simulink model "Vehicle_definitivo_validazione_2"  (R2025b)
settings: Solver=ode4  StartTime=0.0  StopTime=30  FixedStep=0.001  RelTol=1e-3
undefined symbols (not defined in the file): car, new_lotus_bump, new_lotus_roll, new_lotus_steer, posRef, rad, s, Tau_1, Tau_2, Tau_3, Tau_4, yawRef
libraries: aerolibconvert2 x28, simulink_extras x16, simulink x12, slpidlib x2, mpclib x1
(part 13 of 13)

== matlab function Vehicle_definitivo_validazione_2/Senza relaxation/Vehicle/Powertrain/Electric Motor/MATLAB Function ==
  data: T_FR input; T_FL input; w_FR input; w_FL input; SoC input; SoC_dot output
function SoC_dot  = fcn_Battery(T_FR, T_FL, w_FR, w_FL, SoC)
    
    % --- 1. PARAMETRI BATTERIA E POWERTRAIN ---
    C_Ah = 50; % Capacità totale del pacco batteria in Ah (es. accumulatore FS)
    n_cells_series = 100; % Numero di celle collegate in serie
    eta_em = 0.95; % Efficienza combinata Motore + Inverter
    P_aux = 500;   % [Watt] Potenza costantemente assorbita dai servizi (pompe, LV, ECU)
    
    % --- 2. CURVE CARATTERISTICHE (Dipendenti dal SoC) ---
    % Approssimazione lineare per cella Li-ion: da 3.0V (scarica) a 4.2V (carica)
    OCV_cell = 3.0 + (1.2 * SoC); 
    Rin_cell = 0.005; % Resistenza interna della singola cella [Ohm]
    
    V_oc = OCV_cell * n_cells_series; % Tensione a vuoto dell'intero pacco
    R_in = Rin_cell * n_cells_series; % Resistenza interna totale
    
    % --- 3. POTENZA ELETTRICA MOTORE 1 ---
    P_mech1 = T_FR * w_FR;
    if P_mech1 >= 0
        P_elec1 = P_mech1 / eta_em; % Trazione: assorbe più di quanto eroga
    else
        P_elec1 = P_mech1 * eta_em; % Rigenerazione: immette meno di quanto frena
    end
    
    % --- 4. POTENZA ELETTRICA MOTORE 2 ---
    P_mech2 = T_FL * w_FL;
    if P_mech2 >= 0
        P_elec2 = P_mech2 / eta_em; % Trazione
    else
        P_elec2 = P_mech2 * eta_em; % Rigenerazione
    end
    
    % --- 5. CARICO ELETTRICO TOTALE SULLA BATTERIA ---
    % La batteria vede la somma algebrica dei due inverter più i servizi
    P_tot_elec = P_elec1 + P_elec2 + P_aux;
    
    % --- 6. CALCOLO CORRENTE E TENSIONE (CIRCUITO EQUIVALENTE) ---
    % Risoluzione dell'equazione di 2° grado: Rin * I^2 - Voc * I + P_tot = 0
    discriminante = V_oc^2 - 4 * R_in * P_tot_elec;
    
    if discriminante < 0
        % Protezione numerica: la richiesta di potenza supera il limite fisico
        % della batteria (il voltage sag la manderebbe a zero). 
        % Eroga la corrente massima teorica (Cortocircuito).
        I_batt = V_oc / (2 * R_in); 
    else
        % Soluzione standard per la corrente prelevata (o immessa se P_tot < 0)
        I_batt = (V_oc - sqrt(discriminante)) / (2 * R_in);
    end
    
    % Voltaggio reale ai morsetti (al netto del Voltage Sag)
    V_batt = V_oc - R_in * I_batt;
    
    % Potenza dissipata per effetto Joule (utile per dimensionare il raffreddamento)
    P_dissipata = R_in * (I_batt^2);
    
    % --- 7. DERIVATA DELLO STATE OF CHARGE (Coulomb Counting) ---
    % SoC_dot [1/s]. I_batt è in Ampere (C/s), la capacità si porta in Coulomb (*3600)
    SoC_dot = -I_batt / (C_Ah * 3600);
    
end

== matlab function Vehicle_definitivo_validazione_2/Torque Vectoring/Vehicle/Solver/MATLAB Function ==
  data: Fx input; Fy input; toe input; u_dot output size=1; v_dot output size=1; drag input; car input; u input; v input; r input; yaw_rate_dot output size=1; ax output size=1; ay output size=1
function [u_dot, v_dot, yaw_rate_dot, ax, ay]   = fcn_Solver(Fx, Fy, toe, drag, car, u, v, r)

% --- Accelerazione Longitudinale (asse X veicolo) ---
u_dot = ( Fx(1)*cos(toe(1)) - Fy(1)*sin(toe(1)) + ...
          Fx(2)*cos(toe(2)) - Fy(2)*sin(toe(2)) + ...
          Fx(3)*cos(toe(3)) - Fy(3)*sin(toe(3)) + ...
          Fx(4)*cos(toe(4)) - Fy(4)*sin(toe(4)) - drag ) / car.m + v * r;

% --- Accelerazione Laterale (asse Y veicolo) ---
v_dot = ( Fx(1)*sin(toe(1)) + Fy(1)*cos(toe(1)) + ...
          Fx(2)*sin(toe(2)) + Fy(2)*cos(toe(2)) + ...
          Fx(3)*sin(toe(3)) + Fy(3)*cos(toe(3)) + ...
          Fx(4)*sin(toe(4)) + Fy(4)*cos(toe(4)) ) / car.m - u * r;

% --- Derivata del Rateo di Imbardata (attorno asse Z) ---
yaw_rate_dot = 1 / car.Izz * ( ...
    ... % Momento dalle forze laterali all'asse anteriore (+lf)
    (Fx(1)*sin(toe(1)) + Fy(1)*cos(toe(1)) + Fx(2)*sin(toe(2)) + Fy(2)*cos(toe(2))) * car.lf ...
    ... % Momento dalle forze laterali all'asse posteriore (-lr)
  - (Fx(3)*sin(toe(3)) + Fy(3)*cos(toe(3)) + Fx(4)*sin(toe(4)) + Fy(4)*cos(toe(4))) * car.lr ...
   ... % Momento dalla carreggiata anteriore (spinta asimmetrica dx/sx)
  - (Fx(2)*cos(toe(2)) - Fy(2)*sin(toe(2)) - Fx(1)*cos(toe(1)) + Fy(1)*sin(toe(1))) * car.tf / 2 ...
    ... % Momento dalla carreggiata posteriore (spinta asimmetrica dx/sx)
  - (Fx(4)*cos(toe(4)) - Fy(4)*sin(toe(4)) - Fx(3)*cos(toe(3)) + Fy(3)*sin(toe(3))) * car.tr / 2 );

% --- Accelerazioni nel sistema di riferimento ---
ax = u_dot - v * r;
ay = v_dot + u * r;

== matlab function Vehicle_definitivo_validazione_2/Torque Vectoring/Vehicle/Tyres/MATLAB Function ==
  data: Fx input; omega_dot output; Fz input; T_motor input; J input; T_roll input; T_brake_eff input; Rl input
function omega_dot = fcn(Fx, Fz,T_motor, J, T_roll, T_brake_eff, Rl)

omega_dot = zeros(4,1);

    for i=1:4
        if Fz(i) < 10
            omega_dot(i) = T_motor(i) / J(i); 
        else
            omega_dot(i) = (T_motor(i) - T_brake_eff(i) - (Fx(i) * Rl) - T_roll(i)) / J(i);
        end
    end
end

== matlab function Vehicle_definitivo_validazione_2/Torque Vectoring/Vehicle/Tyres/tyres ellisse Adams1 ==
  data: car input; u input; Fx_dot output size=[4 1]; v input; r input; toe input; camber input; tyre_deflection input; Fz input; T_brake input; omega input; Fy_dot output; Fz output; SA output; SR output; T_roll output; T_brake_eff output; Rl output; Fx_dyn input; Fy_dyn input
function [Fx_dot,Fy_dot, Fz,SA,SR,T_roll,T_brake_eff,Rl] = fcn_Tyres(car, u, v, r, toe, camber, tyre_deflection, Fz, T_brake, omega, Fx_dyn, Fy_dyn)
    
    Fx_steady = zeros(4,1);
    Fy_steady = zeros(4,1);
    Fx_dot = zeros(4,1);
    Fy_dot = zeros(4,1);
    SA = zeros(4,1);
    SR = zeros(4,1);    
    T_roll = zeros(4,1);   
    T_brake_eff = zeros(4,1);
            
    % =========================================================
    % 1. CINEMATICA (Calcolo Slip Angle e Velocità)
    % =========================================================
    Vy_F = v + r * car.lf;
    Vy_R = v - r * car.lr;
    
    Vx_FR = u + 0.5 * car.tf * r; 
    Vx_FL = u - 0.5 * car.tf * r; 
    Vx_RR = u + 0.5 * car.tr * r; 
    Vx_RL = u - 0.5 * car.tr * r; 
    Vx = [Vx_FR; Vx_FL; Vx_RR; Vx_RL];
    
    alpha_FR = atan2(Vy_F, Vx_FR);
    alpha_FL = atan2(Vy_F, Vx_FL);
    alpha_RR = atan2(Vy_R, Vx_RR);
    alpha_RL = atan2(Vy_R, Vx_RL);
  
    SA(1) = (toe(1) - alpha_FR);
    SA(2) = (toe(2) - alpha_FL);
    SA(3) = (toe(3) - alpha_RR);
    SA(4) = (toe(4) - alpha_RL);
    SA(isnan(SA)) = 0;
    
    R0 = car.R; % Raggio nominale (indeformato) 
    
    % =========================================================
    % 2. DINAMICA GOMMA E RUOTA (Pacejka Steady-State)
    % =========================================================
    %coefficienti longitudinali
    rbx1 = car.tyre_rbx1; 
    rbx2 = car.tyre_rbx2; 
    rcx1 = car.tyre_rcx1; 
    rex1 = car.tyre_rex1; 
    rex2 = car.tyre_rex2; 
    rhx1 = car.tyre_rhx1; 
    %coefficienti laterali
    rby1 = car.tyre_rby1;  
    rby2 = car.tyre_rby2;  
    rby3 = car.tyre_rby3;  
    rcy1 = car.tyre_rcy1;  
    rey1 = car.tyre_rey1;  
    rey2 = car.tyre_rey2; 
    rhy1 = car.tyre_rhy1;  
    rhy2 = car.tyre_rhy2;  
    rvy1 = car.tyre_rvy1; 
    rvy2 = car.tyre_rvy2;  
    rvy3 = car.tyre_rvy3;  
    rvy4 = car.tyre_rvy4;  
    rvy5 = car.tyre_rvy5;  
    rvy6 = car.tyre_rvy6;

    for i = 1:4
        % --- CALCOLO DEI RAGGI (Metodo Pacejka) ---
        Rl = R0 - tyre_deflection(i); 
        Re = R0 - (tyre_deflection(i) / 3); 
        V_lim = max(abs(Vx(i)), 0.1); 
        SR(i) = (Vx(i) - omega(i) * Re) / V_lim; 
        
        % --- Protezione Decollo Ruota ---
        if Fz(i) < 10
            Fx_dot(i) = 100 * (0 - Fx_dyn(i)); 
            Fy_dot(i) = 100 * (0 - Fy_dyn(i));
             
            T_roll(i) = 0;
            T_brake_eff(i) = T_brake(i) * tanh(omega(i) * 50); 
            continue; 
        end
        
        % --- Estrazione Parametri ---
        Fz0 = car.tyre_Fz0; if Fz0 == 0, Fz0 = max(1, Fz(i)); end
        dfz = (Fz(i) - Fz0)/Fz0;
        pi0 = car.tyre_pi0; dpi = (car.tyre_pressure(i) - pi0)/pi0;
        gamma = camber(i) * pi/180;
        
        % --- Mirroring ---
        Ey3_y = car.tyre_Ey3; Hy1_y = car.tyre_Hy1; Hy2_y = car.tyre_Hy2; 
        Vy1_y = car.tyre_Vy1; Vy2_y = car.tyre_Vy2; gamma_y = gamma;
        if i == 2 || i == 4
            Ey3_y = -Ey3_y; Hy1_y = -Hy1_y; Hy2_y = -Hy2_y;
            Vy1_y = -Vy1_y; Vy2_y = -Vy2_y; gamma_y = -gamma_y; 
        end
        
        % --- A) LATERALE PURO ---
        mu_y = (car.tyre_Dy1 + car.tyre_Dy2*dfz) * (1 - car.tyre_Dy3*(gamma_y^2)) * (1 + car.tyre_py3*dpi + car.tyre_py4*dpi^2) * car.scale_factor;
        mu_y = max(mu_y, 0.05); Dy = mu_y * Fz(i); Cy = car.tyre_Cy1;
        K0_y = car.tyre_Ky1 * Fz0 * (1 + car.tyre_py1*dpi) * sin(2*atan(Fz(i) / (car.tyre_Ky2*Fz0*(1 + car.tyre_py2*dpi))));
        Ky = K0_y * (1 - car.tyre_Ky3*abs(gamma_y)); By = Ky / (Cy*Dy + eps);
        SH_y = Hy1_y + Hy2_y*dfz + car.tyre_Hy3*gamma_y; alpha_eff = -(SA(i) + SH_y);
        Ey = (car.tyre_Ey1 + car.tyre_Ey2*dfz) * (1 - (Ey3_y + car.tyre_Ey4*gamma_y)*sign(alpha_eff)); Ey = min(Ey, 0.999); 
        SVy = Fz(i) * ((Vy1_y + Vy2_y*dfz) + (car.tyre_Vy3 + car.tyre_Vy4*dfz)*gamma_y);
        Fy_pure = Dy * sin(Cy * atan(By*alpha_eff - Ey*(By*alpha_eff - atan(By*alpha_eff))));
        
        % --- B) LONGITUDINALE PURO ---
        mu_x = (car.tyre_Dx1 + car.tyre_Dx2*dfz) * (1 - car.tyre_Dx3*(gamma^2)) * (1 + car.tyre_px3*dpi + car.tyre_px4*dpi^2) * car.scale_factor;
        mu_x = max(mu_x, 0.05); Dx = mu_x * Fz(i); Cx = car.tyre_Cx1;
        Kx = Fz(i) * (car.tyre_Kx1 + car.tyre_Kx2*dfz) * exp(car.tyre_Kx3*dfz) * (1 + car.tyre_px1*dpi + car.tyre_px2*dpi^2); Kx = max(Kx, 0.1); 
        Bx = Kx / (Cx*Dx + eps); SH_x = car.tyre_Hx1 + car.tyre_Hx2*dfz; SR_eff = -(SR(i) + SH_x); 
        Ex = (car.tyre_Ex1 + car.tyre_Ex2*dfz + car.tyre_Ex3*dfz^2) * (1 - car.tyre_Ex4*sign(SR_eff)); Ex = min(Ex, 0.999); 
        SVx = Fz(i) * (car.tyre_Vx1 + car.tyre_Vx2*dfz);
        Fx_pure = Dx * sin(Cx * atan(Bx*SR_eff - Ex*(Bx*SR_eff - atan(Bx*SR_eff))));
        
        %% Calcolo Fx pesata
        SA_s = - (SA(i) + rhx1); 
        Bx_alpha = rbx1 * cos(atan(rbx2 * -SR(i)));
        Cx_alpha = rcx1; 
        Ex_alpha = rex1 + rex2 * dfz;
        %Dx_alpha = Fx_tyres(i) / cos(Cx_alpha * atan((Bx_alpha * rhx1) - Ex_alpha * ((Bx_alpha*  rhx1)-atan(Bx_alpha * rhx1))));    
        Gx = cos(Cx_alpha * atan(Bx_alpha * SA_s - Ex_alpha * (Bx_alpha * SA_s - atan(Bx_alpha * SA_s)))) / cos(Cx_alpha * atan(Bx_alpha * rhx1 - Ex_alpha * (Bx_alpha * rhx1 - atan(Bx_alpha * rhx1))));
        Fx_steady(i) = Fx_pure * Gx;

        %% Calcolo Fy pesata
        SR_s = - (SR(i) + (rhy1 + rhy2 * dfz)); 
        By_k = rby1 * cos(atan(rby2 * (-SA(i) - rby3)));
        Cy_k = rcy1; 
        Ey_k = rey1 + rey2 * dfz;
        %Dy_k = Fy_tyres / cos(Cy_k * atan(By_k * (rhy1 + rhy2 * dfz) - Ey_k * (By_k * (rhy1 + rhy2 * dfz) - atan(By_k * (rhy1 + rhy2 * dfz)))));
        Dy_vk = mu_y * Fz(i) * (rvy1 + rvy2 * dfz + rvy3 * gamma) * cos(atan(rvy4 * -SA(i)));
        Sy_vk = Dy_vk * sin(rvy5 * atan(rvy6 * -SR(i)));
        Gy = cos(Cy_k * atan(By_k * SR_s - Ey_k * (By_k * SR_s - atan(By_k * SR_s)))) / cos(Cy_k * atan(By_k* (rhy1 + rhy2 * dfz) - Ey_k * (By_k * (rhy1 + rhy2 * dfz) - atan(By_k * (rhy1 + rhy2 * dfz)))));
        Fy_steady(i) = Fy_pure * Gy + Sy_vk;
        
        % --- DINAMICA RELAXATION LENGTH ---
        Fx_dot(i) = (V_lim / car.Lx) * (Fx_steady(i) - Fx_dyn(i));
        Fy_dot(i) = (V_lim / car.Ly) * (Fy_steady(i) - Fy_dyn(i));

        % --- E) BILANCIO DINAMICO ALLA RUOTA ---
        T_roll(i) = Fz(i) * car.rolling_resistance * tanh(omega(i) * 10);
        T_brake_eff(i) = T_brake(i) * tanh(omega(i) * 50);  
    end
end

== matlab function Vehicle_definitivo_validazione_2/Torque Vectoring/Vehicle Control Unit/High Level Controller/MATLAB Function ==
  data: u input; steer_volante input; r_target output; car input
function r_target = fcn_ReferenceGenerator(u, steer_volante, car)
 
    L = car.wb0;            
    steering_ratio = 5.0;
    K_us = 0.002;   
    
    delta_ruota = (steer_volante / steering_ratio) * (pi / 180);
    
    if abs(u) < 2.0
        r_target = 0;
    else
        r_target = (u / (L + K_us * (u^2))) * delta_ruota;
    end
    
end

== matlab function Vehicle_definitivo_validazione_2/Torque Vectoring/Vehicle Control Unit/Torque Allocator/MATLAB Function ==
  data: T_req_FR output; Mz_delta input; T_req_FL output; tps_ICE input; bps input; car input
function [T_req_FR, T_req_FL] = fcn_TorqueAllocator(Mz_delta, tps_ICE, bps, car)

    tf = car.tf;           
    R = car.R;             
    tau = car.Tau_EM;      
    
    T_max_motore = 6.5; 
    T_max_regen = 2.5;  
    
    Delta_F = Mz_delta / tf;
    Delta_T_ruota = Delta_F * R;
    Delta_T_motore = Delta_T_ruota / tau; 
    
    if bps > 0
        T_base_motore = - (bps * T_max_regen);
    else
        T_base_motore = tps_ICE * T_max_motore;
    end
    
    T_req_FL = T_base_motore - Delta_T_motore; 
    T_req_FR = T_base_motore + Delta_T_motore; 
    
end

== matlab function Vehicle_definitivo_validazione_2/Con relaxation/Vehicle/Chassis/MATLAB Function4 ==
  data: gear input; car input; Jr_tot output
function Jr_tot  = Jr(gear, car)

if gear == 1 
    Jr_tot = car.Jr_tot_1;
elseif gear == 2 
    Jr_tot = car.Jr_tot_2;
elseif gear == 3 
    Jr_tot = car.Jr_tot_3;
elseif gear == 4
    Jr_tot = car.Jr_tot_4;
else  
    Jr_tot = car.Jr_tot_0;
end

== matlab function Vehicle_definitivo_validazione_2/Con relaxation/Vehicle/Chassis/MATLAB Function5 ==
  data: x input; kin input; ax_prev input; ay_prev input; u input; dx output size=[14 1]; Jr_tot input; F_damp_in input; aero_coeffs input; car input; Fz output size=[4 1]; Drag output size=1; wheel_travel output size=[4 1]; susp_vel_ground output size=[4 1]; IR output size=[4 1]; corner_rh output size=[4 1]; tyre_deflection output; damping output
function [dx, Fz, Drag, wheel_travel, susp_vel_ground, IR, corner_rh, tyre_deflection, damping] = fcn_Ride_Model(x, kin, ax_prev, ay_prev, u, Jr_tot, F_damp_in, aero_coeffs, car)

    % --- 1. Estrazione degli Stati ---
    q  = x(1:7);      % [z_heave; theta_pitch; phi_roll; z_uFL; z_uFR; z_uRL; z_uRR]
    dq = x(8:14);     % Velocità
    damping = x(4);

    % --- 2. UNPACKING PARAMETRI DINAMICI ---  
    IR_FR = car.IR_spring_front;   IR_FL = car.IR_spring_front;
    IR_RR = car.IR_spring_rear;    IR_RL = car.IR_spring_rear;
    tf = car.tf;      tr = car.tr;
    lf = car.lf;      lr = car.lr;
    h_cog = car.h_cog;   
    h_rc_f = car.h_rc_f;    h_rc_r = car.h_rc_r;

    % IR_FR = kin(1);   IR_FL = kin(2);
    % IR_RR = kin(3);    IR_RL = kin(4);
    % 
    % tf = kin(5);      tr = kin(6);
    % lf = kin(7);      lr = kin(8);
    % h_cog = kin(9);   
    % h_rc_f = kin(10);    h_rc_r = kin(11);

    % MEZZE CARREGGIATE
    t_f = tf / 2;
    t_r = tr / 2;

    % --- UNPACKING AERODINAMICA ---
    Cz   = aero_coeffs(1);
    Cx   = aero_coeffs(2);
    x_cp = aero_coeffs(3);

    L = lf + lr;
    g = 9.81;
    ms  = car.m_sprung; Iyy = car.Iyy; Ixx = car.Ixx;
    muf = car.m_unsprung_F; mur = car.m_unsprung_R;

    % --- 3. RIGIDEZZE EQUIVALENTI ALLA RUOTA ---
    IR_f_avg = (IR_FR + IR_FL) / 2;
    IR_r_avg = (IR_RR + IR_RL) / 2;
    IR = [IR_f_avg; IR_f_avg; IR_r_avg; IR_r_avg];

    ksf = car.k_spring_front * 1000 * IR_f_avg^2; 
    ksr = car.k_spring_rear  * 1000 * IR_r_avg^2;  
    ktf = car.k_tyre_front   * 1000; 
    ktr = car.k_tyre_rear    * 1000;

    % Le barre prendono i valori normali. L'approccio esplicito le rende sicure.
    kabf = car.k_ARB_front; 
    kabr = car.k_ARB_rear;  

    % --- 4. CINEMATICA TELAIO (Altezze e Velocità degli attacchi) ---
    z_chassis_FL = q(1) - lf*q(2) + t_f*q(3);
    z_chassis_FR = q(1) - lf*q(2) - t_f*q(3);
    z_chassis_RL = q(1) + lr*q(2) + t_r*q(3);
    z_chassis_RR = q(1) + lr*q(2) - t_r*q(3);

    v_chassis_FL = dq(1) - lf*dq(2) + t_f*dq(3);
    v_chassis_FR = dq(1) - lf*dq(2) - t_f*dq(3);
    v_chassis_RL = dq(1) + lr*dq(2) + t_r*dq(3);
    v_chassis_RR = dq(1) + lr*dq(2) - t_r*dq(3);

    % Corner Ride Heights (Daltezze libere da terra)
    corner_rh = [car.h0_ground_front + z_chassis_FR; 
                 car.h0_ground_front + z_chassis_FL; 
                 car.h0_ground_rear  + z_chassis_RR; 
                 car.h0_ground_rear  + z_chassis_RL];

    % Velocità di compressione ammortizzatore
    susp_vel_ground = [dq(5) - v_chassis_FR; 
                       dq(4) - v_chassis_FL; 
                       dq(7) - v_chassis_RR; 
                       dq(6) - v_chassis_RL];

    % --- 5. COMPRESSIONE SOSPENSIONI ---
    % delta_z: compressione della sospensione (Positivo = ruota più vicina al telaio)
    delta_z_FL = q(4) - z_chassis_FL;
    delta_z_FR = q(5) - z_chassis_FR;
    delta_z_RL = q(6) - z_chassis_RL;
    delta_z_RR = q(7) - z_chassis_RR;

    % --- 6. FORZE SOSPENSIONI ---
    % 1. Forze Molle
    F_spring_FL = ksf * delta_z_FL;
    F_spring_FR = ksf * delta_z_FR;
    F_spring_RL = ksr * delta_z_RL;
    F_spring_RR = ksr * delta_z_RR;

    % 2. Forze Barre Antirollio (Differenza di compressione sullo stesso asse)
    F_arb_FL = kabf * (delta_z_FL - delta_z_FR);
    F_arb_FR = kabf * (delta_z_FR - delta_z_FL);
    F_arb_RL = kabr * (delta_z_RL - delta_z_RR);
    F_arb_RR = kabr * (delta_z_RR - delta_z_RL);

    % 3. Forze Damper (Input dalla tua lookup table)
    F_d_FR = F_damp_in(1);
    F_d_FL = F_damp_in(2);
    F_d_RR = F_damp_in(3);
    F_d_RL = F_damp_in(4);

    % FORZA TOTALE DELLA SOSPENSIONE SUL TELAIO
    F_susp_FL = F_spring_FL + F_arb_FL + F_d_FL;
    F_susp_FR = F_spring_FR + F_arb_FR + F_d_FR;
    F_susp_RL = F_spring_RL + F_arb_RL + F_d_RL;
    F_susp_RR = F_spring_RR + F_arb_RR + F_d_RR;

    % --- 7. FORZANTI ESTERNE ---
    Downforce = 0.5 * car.rho * car.frontal_area * Cz * (u^2);
    Drag      = 0.5 * car.rho * car.frontal_area * Cx * (u^2);

    M_aero_pitch = -Drag * (car.h_cp - h_cog) + Downforce * (lf - x_cp);
    M_pitch_ext  = -(car.m * ax_prev * h_cog) + M_aero_pitch;

    h_rc = (h_rc_f * lr + h_rc_r * lf) / L;
    M_roll_ext   = (car.m * ay_prev * (h_cog - h_rc));

    % --- 8. RISOLUZIONE MODELLO (EQUAZIONI DIFFERENZIALI) ---
    % A. MASSA SOSPESA (Telaio)
    sum_Fz_chassis = F_susp_FL + F_susp_FR + F_susp_RL + F_susp_RR - Downforce;
    sum_M_pitch    = -(F_susp_FL + F_susp_FR)*lf + (F_susp_RL + F_susp_RR)*lr + M_pitch_ext;
    sum_M_roll     =  (F_susp_FL - F_susp_FR)*t_f + (F_susp_RL - F_susp_RR)*t_r + M_roll_ext;

    ddq_heave = sum_Fz_chassis / ms;
    ddq_pitch = sum_M_pitch / Iyy;
    ddq_roll  = sum_M_roll / Ixx;

    % B. MASSE NON SOSPESE (Ruote)
    % La gomma spinge la ruota verso l'alto
    F_tyre_FL = -ktf * q(4);
    F_tyre_FR = -ktf * q(5);
    F_tyre_RL = -ktr * q(6);
    F_tyre_RR = -ktr * q(7);

    % La sospensione spinge la ruota in verso opposto rispetto a come spinge il telaio
    ddq_uFL = (F_tyre_FL - F_susp_FL) / muf;
    ddq_uFR = (F_tyre_FR - F_susp_FR) / muf;
    ddq_uRL = (F_tyre_RL - F_susp_RL) / mur;
    ddq_uRR = (F_tyre_RR - F_susp_RR) / mur;

    % Ricompattamento
    ddq = [ddq_heave; ddq_pitch; ddq_roll; ddq_uFL; ddq_uFR; ddq_uRL; ddq_uRR];
    dx  = [dq; ddq];

    % --- 9. CALCOLO FZ A TERRA ---
    delta_Fz_geom_front = (car.m * ay_prev * (lr / L) * h_rc_f) / tf;
    delta_Fz_geom_rear  = (car.m * ay_prev * (lf / L) * h_rc_r) / tr;

    delta_Fz_inertia  = (2 * Jr_tot + 2 * car.J_f) * ax_prev / (car.R * L);
    delta_Fz_roll_res = (car.m * g + Downforce) * car.rolling_resistance / L;

    Fz_stat_f = (car.m * g * lr / L) / 2;
    Fz_stat_r = (car.m * g * lf / L) / 2;

    Fz_FR = Fz_stat_f - ktf * q(5) + delta_Fz_geom_front - delta_Fz_inertia - delta_Fz_roll_res; 
    Fz_FL = Fz_stat_f - ktf * q(4) - delta_Fz_geom_front - delta_Fz_inertia - delta_Fz_roll_res; 
    Fz_RR = Fz_stat_r - ktr * q(7) + delta_Fz_geom_rear  + delta_Fz_inertia + delta_Fz_roll_res; 
    Fz_RL = Fz_stat_r - ktr * q(6) - delta_Fz_geom_rear  + delta_Fz_inertia + delta_Fz_roll_res; 

    Fz = [Fz_FR; Fz_FL; Fz_RR; Fz_RL];
    Fz(Fz < 0) = 0; 

    % --- 10. OUTPUT CINEMATICI FINALI (Con Virtual Rails) ---

    wheel_travel = [delta_z_FR; 
                    delta_z_FL; 
                    delta_z_RR; 
                    delta_z_RL] * 1000; 
    
    tyre_deflection = [Fz(1) / ktf;
                       Fz(2) / ktf;
                       Fz(3) / ktr;
                       Fz(4) / ktr];
end

== matlab function Vehicle_definitivo_validazione_2/Senza relaxation/Vehicle/Powertrain/pwt con clutch/Differential1 ==
  data: T_rear input; T_RR output; w_RR input; w_RL input; T_RL output; car input
function [T_RR, T_RL] = fcn_Salisbury_LSD(T_rear, w_RR, w_RL, car)
   
    % Coefficienti di smoothing (Stabilità Simulink)
    k_blend = 10; 
    k_slip  = 5; 
    
    % --- 2. TRANSIZIONE POWER-ON / POWER-OFF (Senza IF) ---
    w_blend = 0.5 * (1 + tanh(k_blend * T_rear));
    mu_active = car.mu_Poff + (car.mu_Pon - car.mu_Poff) * w_blend;
    
    % --- 3. CALCOLO CAPACITÀ DI BLOCCAGGIO (Mf_max) ---
    T_ramps = mu_active * abs(T_rear);
    Mf_max = max(car.Mf_preload, T_ramps); 
    
    % --- 4. APPLICAZIONE COPPIA ATTRITO (Modello Continuo) ---
    delta_w = w_RR - w_RL; 
    T_lock = Mf_max * tanh(k_slip * delta_w);
    
    % --- 5. RIPARTIZIONE FINALE ---
    % Se w_RR è maggiore (delta_w > 0, T_lock > 0), tolgo a RR e do a RL
    T_RR = (T_rear / 2) - T_lock;
    T_RL = (T_rear / 2) + T_lock;
end

== matlab function Vehicle_definitivo_validazione_2/Con relaxation/Vehicle/Powertrain/Electric Motor/MATLAB Function ==
  data: T_FR input; T_FL input; w_FR input; w_FL input; SoC input; SoC_dot output
function SoC_dot  = fcn_Battery(T_FR, T_FL, w_FR, w_FL, SoC)
    
    % --- 1. PARAMETRI BATTERIA E POWERTRAIN ---
    C_Ah = 50; % Capacità totale del pacco batteria in Ah (es. accumulatore FS)
    n_cells_series = 100; % Numero di celle collegate in serie
    eta_em = 0.95; % Efficienza combinata Motore + Inverter
    P_aux = 500;   % [Watt] Potenza costantemente assorbita dai servizi (pompe, LV, ECU)
    
    % --- 2. CURVE CARATTERISTICHE (Dipendenti dal SoC) ---
    % Approssimazione lineare per cella Li-ion: da 3.0V (scarica) a 4.2V (carica)
    OCV_cell = 3.0 + (1.2 * SoC); 
    Rin_cell = 0.005; % Resistenza interna della singola cella [Ohm]
    
    V_oc = OCV_cell * n_cells_series; % Tensione a vuoto dell'intero pacco
    R_in = Rin_cell * n_cells_series; % Resistenza interna totale
    
    % --- 3. POTENZA ELETTRICA MOTORE 1 ---
    P_mech1 = T_FR * w_FR;
    if P_mech1 >= 0
        P_elec1 = P_mech1 / eta_em; % Trazione: assorbe più di quanto eroga
    else
        P_elec1 = P_mech1 * eta_em; % Rigenerazione: immette meno di quanto frena
    end
    
    % --- 4. POTENZA ELETTRICA MOTORE 2 ---
    P_mech2 = T_FL * w_FL;
    if P_mech2 >= 0
        P_elec2 = P_mech2 / eta_em; % Trazione
    else
        P_elec2 = P_mech2 * eta_em; % Rigenerazione
    end
    
    % --- 5. CARICO ELETTRICO TOTALE SULLA BATTERIA ---
    % La batteria vede la somma algebrica dei due inverter più i servizi
    P_tot_elec = P_elec1 + P_elec2 + P_aux;
    
    % --- 6. CALCOLO CORRENTE E TENSIONE (CIRCUITO EQUIVALENTE) ---
    % Risoluzione dell'equazione di 2° grado: Rin * I^2 - Voc * I + P_tot = 0
    discriminante = V_oc^2 - 4 * R_in * P_tot_elec;
    
    if discriminante < 0
        % Protezione numerica: la richiesta di potenza supera il limite fisico
        % della batteria (il voltage sag la manderebbe a zero). 
        % Eroga la corrente massima teorica (Cortocircuito).
        I_batt = V_oc / (2 * R_in); 
    else
        % Soluzione standard per la corrente prelevata (o immessa se P_tot < 0)
        I_batt = (V_oc - sqrt(discriminante)) / (2 * R_in);
    end
    
    % Voltaggio reale ai morsetti (al netto del Voltage Sag)
    V_batt = V_oc - R_in * I_batt;
    
    % Potenza dissipata per effetto Joule (utile per dimensionare il raffreddamento)
    P_dissipata = R_in * (I_batt^2);
    
    % --- 7. DERIVATA DELLO STATE OF CHARGE (Coulomb Counting) ---
    % SoC_dot [1/s]. I_batt è in Ampere (C/s), la capacità si porta in Coulomb (*3600)
    SoC_dot = -I_batt / (C_Ah * 3600);
    
end

== matlab function Vehicle_definitivo_validazione_2/Con relaxation/Vehicle/Powertrain/pwt con clutch/MATLAB Function1 ==
  data: w_ice input; condizione output; w_rear input
function condizione = fcn(w_ice, w_rear)
    
if (w_ice - w_rear) < 50
    condizione = true;
else
    condizione = false;
end

end

== matlab function Vehicle_definitivo_validazione_2/Con relaxation/Vehicle/Powertrain/pwt con clutch/MATLAB Function4 ==
  data: u input; next_gear output; tps input; bps input; current_gear input; shift_timer_in input; shift_timer_out output; torque_mult output
function [next_gear, shift_timer_out, torque_mult] = Gearbox_ECU(u, tps, bps, current_gear, shift_timer_in)
   
    dt = 0.001;               
    shift_duration = 0.030;   
    nGearMax = 4;             
    
    v_thresh_up   = [0, 24.9444, 29.1, inf]; 
    v_thresh_down = [0, 18, 26.5, 29.5];
    
    % Inizializzazione sicura
    % if current_gear == 0
    %     current_gear = 2; % Partenza in 2° marcia
    % end
    
    next_gear = current_gear;
    
    if shift_timer_in > 0
        torque_mult = 0;                           
        shift_timer_out = shift_timer_in - dt;     
    else
        torque_mult = 1;                           
        shift_timer_out = 0;                       
        if current_gear < nGearMax && u >= v_thresh_up(current_gear) && tps > 0 && bps == 0
            next_gear = current_gear + 1;
            shift_timer_out = shift_duration;                  
        elseif current_gear > 1 && u <= v_thresh_down(current_gear) && (bps > 0 || tps == 0)
            next_gear = current_gear - 1;
            shift_timer_out = shift_duration;      
        end
    end
end

== matlab function Vehicle_definitivo_validazione_2/Con relaxation/Vehicle/Powertrain/pwt senza clutch/Differential ==
  data: T_rear input; T_RR output; w_RR input; w_RL input; T_RL output; car input
function [T_RR, T_RL] = fcn_Salisbury_LSD(T_rear, w_RR, w_RL, car)
   
    % Coefficienti di smoothing (Stabilità Simulink)
    k_blend = 10; 
    k_slip  = 5; 
    
    % --- 2. TRANSIZIONE POWER-ON / POWER-OFF (Senza IF) ---
    w_blend = 0.5 * (1 + tanh(k_blend * T_rear));
    mu_active = car.mu_Poff + (car.mu_Pon - car.mu_Poff) * w_blend;
    
    % --- 3. CALCOLO CAPACITÀ DI BLOCCAGGIO (Mf_max) ---
    T_ramps = mu_active * abs(T_rear);
    Mf_max = max(car.Mf_preload, T_ramps); 
    
    % --- 4. APPLICAZIONE COPPIA ATTRITO (Modello Continuo) ---
    delta_w = w_RR - w_RL; 
    T_lock = Mf_max * tanh(k_slip * delta_w);
    
    % --- 5. RIPARTIZIONE FINALE ---
    % Se w_RR è maggiore (delta_w > 0, T_lock > 0), tolgo a RR e do a RL
    T_RR = (T_rear / 2) - T_lock;
    T_RL = (T_rear / 2) + T_lock;
end

== matlab function Vehicle_definitivo_validazione_2/Con relaxation/Vehicle/Powertrain/pwt senza clutch/Gearbox ==
  data: u input; next_gear output; torque_mult output; tps input; bps input; current_gear input; shift_timer_in input; shift_timer_out output
function [next_gear, torque_mult, shift_timer_out] = Gearbox_ECU(u, tps, bps, current_gear, shift_timer_in)
   
    dt = 0.001;               
    shift_duration = 0.030;   
    nGearMax = 4;             
    
    v_thresh_up   = [0, 24.9444, 29.1, inf]; 
    v_thresh_down = [0, 18, 26.5, 29.5];
    
    % Inizializzazione sicura
    % if current_gear == 0
    %     current_gear = 2; % Partenza in 2° marcia
    % end
    
    next_gear = current_gear;
    
    if shift_timer_in > 0
        torque_mult = 0;                           
        shift_timer_out = shift_timer_in - dt;     
    else
        torque_mult = 1;                           
        shift_timer_out = 0;                       
        if current_gear < nGearMax && u >= v_thresh_up(current_gear) && tps > 0 && bps == 0
            next_gear = current_gear + 1;
            shift_timer_out = shift_duration;                  
        elseif current_gear > 1 && u <= v_thresh_down(current_gear) && (bps > 0 || tps == 0)
            next_gear = current_gear - 1;
            shift_timer_out = shift_duration;      
        end
    end
end

== matlab function Vehicle_definitivo_validazione_2/Con relaxation/Vehicle/Solver/MATLAB Function ==
  data: Fx input; Fy input; toe input; u_dot output size=1; v_dot output size=1; drag input; car input; u input; v input; r input; yaw_rate_dot output size=1; ax output size=1; ay output size=1
function [u_dot, v_dot, yaw_rate_dot, ax, ay]   = fcn_Solver(Fx, Fy, toe, drag, car, u, v, r)

% --- Accelerazione Longitudinale (asse X veicolo) ---
u_dot = ( Fx(1)*cos(toe(1)) - Fy(1)*sin(toe(1)) + ...
          Fx(2)*cos(toe(2)) - Fy(2)*sin(toe(2)) + ...
          Fx(3)*cos(toe(3)) - Fy(3)*sin(toe(3)) + ...
          Fx(4)*cos(toe(4)) - Fy(4)*sin(toe(4)) - drag ) / car.m + v * r;

% --- Accelerazione Laterale (asse Y veicolo) ---
v_dot = ( Fx(1)*sin(toe(1)) + Fy(1)*cos(toe(1)) + ...
          Fx(2)*sin(toe(2)) + Fy(2)*cos(toe(2)) + ...
          Fx(3)*sin(toe(3)) + Fy(3)*cos(toe(3)) + ...
          Fx(4)*sin(toe(4)) + Fy(4)*cos(toe(4)) ) / car.m - u * r;

% --- Derivata del Rateo di Imbardata (attorno asse Z) ---
yaw_rate_dot = 1 / car.Izz * ( ...
    ... % Momento dalle forze laterali all'asse anteriore (+lf)
    (Fx(1)*sin(toe(1)) + Fy(1)*cos(toe(1)) + Fx(2)*sin(toe(2)) + Fy(2)*cos(toe(2))) * car.lf ...
    ... % Momento dalle forze laterali all'asse posteriore (-lr)
  - (Fx(3)*sin(toe(3)) + Fy(3)*cos(toe(3)) + Fx(4)*sin(toe(4)) + Fy(4)*cos(toe(4))) * car.lr ...
   ... % Momento dalla carreggiata anteriore (spinta asimmetrica dx/sx)
  - (Fx(2)*cos(toe(2)) - Fy(2)*sin(toe(2)) - Fx(1)*cos(toe(1)) + Fy(1)*sin(toe(1))) * car.tf / 2 ...
    ... % Momento dalla carreggiata posteriore (spinta asimmetrica dx/sx)
  - (Fx(4)*cos(toe(4)) - Fy(4)*sin(toe(4)) - Fx(3)*cos(toe(3)) + Fy(3)*sin(toe(3))) * car.tr / 2 );

% --- Accelerazioni nel sistema di riferimento ---
ax = u_dot - v * r;
ay = v_dot + u * r;

== matlab function Vehicle_definitivo_validazione_2/Con relaxation/Vehicle/Tyres/MATLAB Function ==
  data: Fx input; omega_dot output; Fz input; T_motor input; J input; T_roll input; T_brake_eff input; Rl input
function omega_dot = fcn(Fx, Fz,T_motor, J, T_roll, T_brake_eff, Rl)

omega_dot = zeros(4,1);

    for i=1:4
        if Fz(i) < 10
            omega_dot(i) = T_motor(i) / J(i); 
        else
            omega_dot(i) = (T_motor(i) - T_brake_eff(i) - (Fx(i) * Rl) - T_roll(i)) / J(i);
        end
    end
end

== matlab function Vehicle_definitivo_validazione_2/Con relaxation/Vehicle/Tyres/tyres ellisse Adams1 ==
  data: car input; u input; Fx_dot output size=[4 1]; v input; r input; toe input; camber input; tyre_deflection input; Fz input; T_brake input; omega input; Fy_dot output; Fz output; SA output; SR output; T_roll output; T_brake_eff output; Rl output; Fx_dyn input; Fy_dyn input
function [Fx_dot,Fy_dot, Fz,SA,SR,T_roll,T_brake_eff,Rl] = fcn_Tyres(car, u, v, r, toe, camber, tyre_deflection, Fz, T_brake, omega, Fx_dyn, Fy_dyn)
    
    Fx_steady = zeros(4,1);
    Fy_steady = zeros(4,1);
    Fx_dot = zeros(4,1);
    Fy_dot = zeros(4,1);
    SA = zeros(4,1);
    SR = zeros(4,1);    
    T_roll = zeros(4,1);   
    T_brake_eff = zeros(4,1);
            
    % =========================================================
    % 1. CINEMATICA (Calcolo Slip Angle e Velocità)
    % =========================================================
    Vy_F = v + r * car.lf;
    Vy_R = v - r * car.lr;
    
    Vx_FR = u + 0.5 * car.tf * r; 
    Vx_FL = u - 0.5 * car.tf * r; 
    Vx_RR = u + 0.5 * car.tr * r; 
    Vx_RL = u - 0.5 * car.tr * r; 
    Vx = [Vx_FR; Vx_FL; Vx_RR; Vx_RL];
    
    alpha_FR = atan2(Vy_F, Vx_FR);
    alpha_FL = atan2(Vy_F, Vx_FL);
    alpha_RR = atan2(Vy_R, Vx_RR);
    alpha_RL = atan2(Vy_R, Vx_RL);
  
    SA(1) = (toe(1) - alpha_FR);
    SA(2) = (toe(2) - alpha_FL);
    SA(3) = (toe(3) - alpha_RR);
    SA(4) = (toe(4) - alpha_RL);
    SA(isnan(SA)) = 0;
    
    R0 = car.R; % Raggio nominale (indeformato) 
    
    % =========================================================
    % 2. DINAMICA GOMMA E RUOTA (Pacejka Steady-State)
    % =========================================================
    %coefficienti longitudinali
    rbx1 = car.tyre_rbx1; 
    rbx2 = car.tyre_rbx2; 
    rcx1 = car.tyre_rcx1; 
    rex1 = car.tyre_rex1; 
    rex2 = car.tyre_rex2; 
    rhx1 = car.tyre_rhx1; 
    %coefficienti laterali
    rby1 = car.tyre_rby1;  
    rby2 = car.tyre_rby2;  
    rby3 = car.tyre_rby3;  
    rcy1 = car.tyre_rcy1;  
    rey1 = car.tyre_rey1;  
    rey2 = car.tyre_rey2; 
    rhy1 = car.tyre_rhy1;  
    rhy2 = car.tyre_rhy2;  
    rvy1 = car.tyre_rvy1; 
    rvy2 = car.tyre_rvy2;  
    rvy3 = car.tyre_rvy3;  
    rvy4 = car.tyre_rvy4;  
    rvy5 = car.tyre_rvy5;  
    rvy6 = car.tyre_rvy6;

    for i = 1:4
        % --- CALCOLO DEI RAGGI (Metodo Pacejka) ---
        Rl = R0 - tyre_deflection(i); 
        Re = R0 - (tyre_deflection(i) / 3); 
        V_lim = max(abs(Vx(i)), 0.1); 
        SR(i) = (Vx(i) - omega(i) * Re) / V_lim; 
        
        % --- Protezione Decollo Ruota ---
        if Fz(i) < 10
            Fx_dot(i) = 100 * (0 - Fx_dyn(i)); 
            Fy_dot(i) = 100 * (0 - Fy_dyn(i));
             
            T_roll(i) = 0;
            T_brake_eff(i) = T_brake(i) * tanh(omega(i) * 50); 
            continue; 
        end
        
        % --- Estrazione Parametri ---
        Fz0 = car.tyre_Fz0; if Fz0 == 0, Fz0 = max(1, Fz(i)); end
        dfz = (Fz(i) - Fz0)/Fz0;
        pi0 = car.tyre_pi0; dpi = (car.tyre_pressure(i) - pi0)/pi0;
        gamma = camber(i) * pi/180;
        
        % --- Mirroring ---
        Ey3_y = car.tyre_Ey3; Hy1_y = car.tyre_Hy1; Hy2_y = car.tyre_Hy2; 
        Vy1_y = car.tyre_Vy1; Vy2_y = car.tyre_Vy2; gamma_y = gamma;
        if i == 2 || i == 4
            Ey3_y = -Ey3_y; Hy1_y = -Hy1_y; Hy2_y = -Hy2_y;
            Vy1_y = -Vy1_y; Vy2_y = -Vy2_y; gamma_y = -gamma_y; 
        end
        
        % --- A) LATERALE PURO ---
        mu_y = (car.tyre_Dy1 + car.tyre_Dy2*dfz) * (1 - car.tyre_Dy3*(gamma_y^2)) * (1 + car.tyre_py3*dpi + car.tyre_py4*dpi^2) * car.scale_factor;
        mu_y = max(mu_y, 0.05); Dy = mu_y * Fz(i); Cy = car.tyre_Cy1;
        K0_y = car.tyre_Ky1 * Fz0 * (1 + car.tyre_py1*dpi) * sin(2*atan(Fz(i) / (car.tyre_Ky2*Fz0*(1 + car.tyre_py2*dpi))));
        Ky = K0_y * (1 - car.tyre_Ky3*abs(gamma_y)); By = Ky / (Cy*Dy + eps);
        SH_y = Hy1_y + Hy2_y*dfz + car.tyre_Hy3*gamma_y; alpha_eff = -(SA(i) + SH_y);
        Ey = (car.tyre_Ey1 + car.tyre_Ey2*dfz) * (1 - (Ey3_y + car.tyre_Ey4*gamma_y)*sign(alpha_eff)); Ey = min(Ey, 0.999); 
        SVy = Fz(i) * ((Vy1_y + Vy2_y*dfz) + (car.tyre_Vy3 + car.tyre_Vy4*dfz)*gamma_y);
        Fy_pure = Dy * sin(Cy * atan(By*alpha_eff - Ey*(By*alpha_eff - atan(By*alpha_eff))));
        
        % --- B) LONGITUDINALE PURO ---
        mu_x = (car.tyre_Dx1 + car.tyre_Dx2*dfz) * (1 - car.tyre_Dx3*(gamma^2)) * (1 + car.tyre_px3*dpi + car.tyre_px4*dpi^2) * car.scale_factor;
        mu_x = max(mu_x, 0.05); Dx = mu_x * Fz(i); Cx = car.tyre_Cx1;
        Kx = Fz(i) * (car.tyre_Kx1 + car.tyre_Kx2*dfz) * exp(car.tyre_Kx3*dfz) * (1 + car.tyre_px1*dpi + car.tyre_px2*dpi^2); Kx = max(Kx, 0.1); 
        Bx = Kx / (Cx*Dx + eps); SH_x = car.tyre_Hx1 + car.tyre_Hx2*dfz; SR_eff = -(SR(i) + SH_x); 
        Ex = (car.tyre_Ex1 + car.tyre_Ex2*dfz + car.tyre_Ex3*dfz^2) * (1 - car.tyre_Ex4*sign(SR_eff)); Ex = min(Ex, 0.999); 
        SVx = Fz(i) * (car.tyre_Vx1 + car.tyre_Vx2*dfz);
        Fx_pure = Dx * sin(Cx * atan(Bx*SR_eff - Ex*(Bx*SR_eff - atan(Bx*SR_eff))));
        
        %% Calcolo Fx pesata
        SA_s = - (SA(i) + rhx1); 
        Bx_alpha = rbx1 * cos(atan(rbx2 * -SR(i)));
        Cx_alpha = rcx1; 
        Ex_alpha = rex1 + rex2 * dfz;
        %Dx_alpha = Fx_tyres(i) / cos(Cx_alpha * atan((Bx_alpha * rhx1) - Ex_alpha * ((Bx_alpha*  rhx1)-atan(Bx_alpha * rhx1))));    
        Gx = cos(Cx_alpha * atan(Bx_alpha * SA_s - Ex_alpha * (Bx_alpha * SA_s - atan(Bx_alpha * SA_s)))) / cos(Cx_alpha * atan(Bx_alpha * rhx1 - Ex_alpha * (Bx_alpha * rhx1 - atan(Bx_alpha * rhx1))));
        Fx_steady(i) = Fx_pure * Gx;

        %% Calcolo Fy pesata
        SR_s = - (SR(i) + (rhy1 + rhy2 * dfz)); 
        By_k = rby1 * cos(atan(rby2 * (-SA(i) - rby3)));
        Cy_k = rcy1; 
        Ey_k = rey1 + rey2 * dfz;
        %Dy_k = Fy_tyres / cos(Cy_k * atan(By_k * (rhy1 + rhy2 * dfz) - Ey_k * (By_k * (rhy1 + rhy2 * dfz) - atan(By_k * (rhy1 + rhy2 * dfz)))));
        Dy_vk = mu_y * Fz(i) * (rvy1 + rvy2 * dfz + rvy3 * gamma) * cos(atan(rvy4 * -SA(i)));
        Sy_vk = Dy_vk * sin(rvy5 * atan(rvy6 * -SR(i)));
        Gy = cos(Cy_k * atan(By_k * SR_s - Ey_k * (By_k * SR_s - atan(By_k * SR_s)))) / cos(Cy_k * atan(By_k* (rhy1 + rhy2 * dfz) - Ey_k * (By_k * (rhy1 + rhy2 * dfz) - atan(By_k * (rhy1 + rhy2 * dfz)))));
        Fy_steady(i) = Fy_pure * Gy + Sy_vk;
        
        % --- DINAMICA RELAXATION LENGTH ---
        Fx_dot(i) = (V_lim / car.Lx) * (Fx_steady(i) - Fx_dyn(i));
        Fy_dot(i) = (V_lim / car.Ly) * (Fy_steady(i) - Fy_dyn(i));

        % --- E) BILANCIO DINAMICO ALLA RUOTA ---
        T_roll(i) = Fz(i) * car.rolling_resistance * tanh(omega(i) * 10);
        T_brake_eff(i) = T_brake(i) * tanh(omega(i) * 50);  
    end
end

== matlab function Vehicle_definitivo_validazione_2/Senza relaxation/Vehicle/Powertrain/pwt con clutch/MATLAB Function1 ==
  data: w_ice input; condizione output; w_rear input
function condizione = fcn(w_ice, w_rear)
    
if (w_ice - w_rear) < 50
    condizione = true;
else
    condizione = false;
end

end
